simulink model "AGTF30_eng"  (Simulink 8.5)
settings: Solver=FixedStepDiscrete  StartTime=0.0  StopTime=10.0  FixedStep=0.015  RelTol=1e-3  SampleTimeConstraint=STIndependent
model workspace: external: MAT-File (data not in the file)
undefined symbols (not defined in the file or in its folder): MWS, stripchar_TMATS
libraries: Lib_Turbo_StaticCalc_TMATS x6, Lib_Turbo_Compressor_TMATS x3, Lib_Turbo_TurbineNPSS_TMATS x2, Lib_Turbo_Shaft_TMATS x2, Lib_Turbo_Ambient_TMATS x1, Lib_Turbo_Nozzle_TMATS x1, Lib_Turbo_NozzleVar_TMATS x1, Lib_Turbo_Burner_TMATS x1, Lib_Solve_DataOut_TMATS x1, Lib_Turbo_GearBox_TMATS x1, Lib_Turbo_Inlet_TMATS x1, Lib_Turbo_Splitter_TMATS x1
settings Model: Creator=jwchapm2  LastModifiedBy=jwchapm2
settings DataIOCC: ExternalInput=[0 0]  InitialState=[]  SignalLoggingSaveFormat=Dataset  SaveOutput=off  SignalLogging=off  DSMLogging=off  SaveTime=off
settings OptimizationCC: InlineParams=on  BufferReuse=off  ExpressionDepthLimit=128
settings DebuggingCC: UnderspecifiedInitializationDetection=Simplified  MergeDetectMultiDrivingBlocksExec=error  FcnCallInpInsideContextMsg=EnableAllAsError  StateNameClashWarn=none  InitInArrayFormatMsg=none
settings ModelReferenceCC: ModelReferenceNumInstancesAllowed=Single
settings GRTTargetCC: CombineOutputUpdateFcns=on  GRTInterface=off

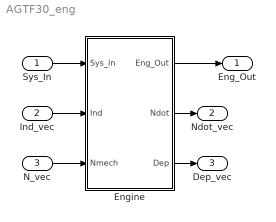
== system AGTF30_eng ==
  Sys_In : Inport
  Ind_vec : Inport  Port=2
  N_vec : Inport  Port=3
  Engine : Subsystem
  Eng_Out : Outport  OutDataTypeStr=Bus: Eng_Bus
  Ndot_vec : Outport  Port=2
  Dep_vec : Outport  Port=3
  wires:
  Sys_In/1 -> Engine/1(Sys_In)
  N_vec/1 -> Engine/3(Nmech)
  Ind_vec/1 -> Engine/2(Ind)
  Engine/3(Dep) -> Dep_vec/1
  Engine/2(Ndot) -> Ndot_vec/1
  Engine/1(Eng_Out) -> Eng_Out/1

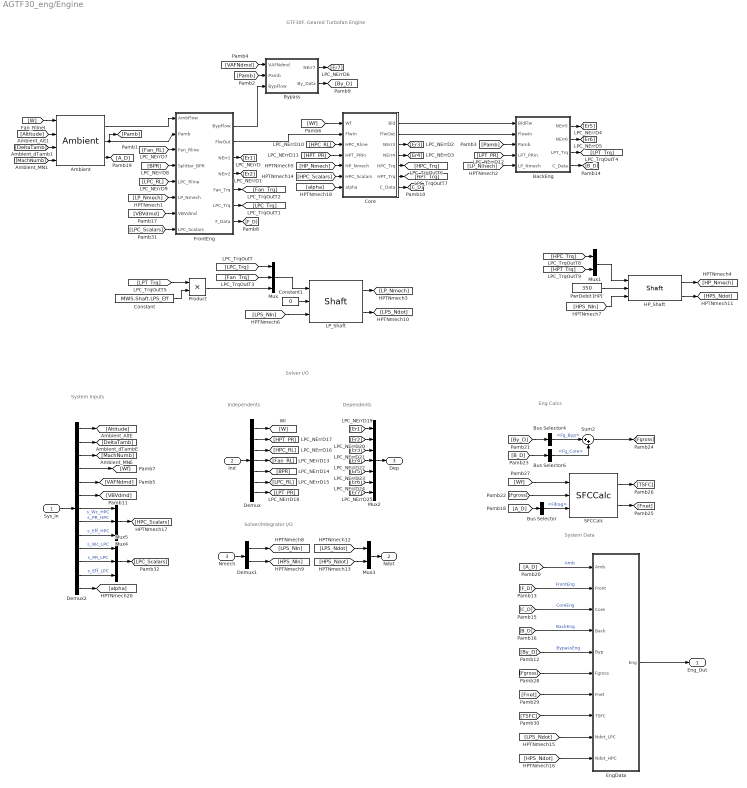
== system AGTF30_eng/Engine ==
  note: GTF30F, Geared Turbofan Engine
  note: System Inputs
  note: Solver I/O
  note: System Data
  note: Solver/Integrator I/O
  note: Independents
  note: Dependents
  note: Eng Calcs
  Sys_In : Inport
  Ind : Inport  Port=2
  Nmech : Inport  Port=3
  Ambient : Lib_Turbo_Ambient_TMATS/Ambient  X_A_AltVec_M=5000*[-1 0 1 2 3 4 5 6 7 8 9 10 12 14 16]  T_A_TsVec_M=[536.51 518.67 500.84 483.03 465.22 447.41 429.62 411.84 394.06 389.97 389.97 389.97 389.97 392.25 397.69]  T_A_PsVec_M=[17.554 14.696 12.228 10.108 8.297 6.759 5.461 4.373 3.468 2.73 2.149 1.692 1.049 0.651 0.406]  AFARc_M=0  X_A_FARVec_M=[0; 0.0050; 0.0100; 0.0150; 0.0200; 0.0250; 0.0300]  T_A_RtArray_M="[0.0686;    0.0686;    0.0686;    0.0686;    0.0686;    0.0686;    0.0686]"  Y_A_TVec_M=[300 10000]  T_A_gammaArray_M=[ 1.4 1.4 1.4 1.4 1.4 1.4 1.4; 1.4 1.4 1.4 1.4 1.4 1.4 1.4]
  BackEng : Subsystem
  Bus Selector : BusSelector  OutputSignals=Fdrag
  Bus Selector4 : BusSelector  OutputSignals=Fg_Byp
  Bus Selector6 : BusSelector  OutputSignals=Fg_Core
  Bypass : Subsystem
  Constant : Constant  Value=MWS.Shaft.LPS_Eff
  Constant1 : Constant  Value=0
  Core : Subsystem
  Demux : Demux  Outputs=7
  Demux1 : Demux  Outputs=2
  Demux2 : Demux  Outputs=13
  EngData : Subsystem
  FrontEng : Subsystem
  HP_Shaft : Lib_Turbo_Shaft_TMATS/Shaft  Shaft_Inertia_M=MWS.Shaft.HPS_Inertia
  LP_Shaft : Lib_Turbo_Shaft_TMATS/Shaft  Shaft_Inertia_M=MWS.Shaft.LPS_Inertia
  Mux : Mux  Inputs=3
  Mux1 : Mux  Inputs=2
  Mux2 : Mux  Inputs=7
  Mux3 : Mux  Inputs=2
  Mux4 : Mux  Inputs=3
  Mux5 : Mux  Inputs=3
  Product : Product
  PwrDebit [HP] : Constant  Value=350
  SFCCalc : Lib_Turbo_SFCCalc_TMATS/SFCCalc
  Sum2 : Sum  Inputs=|++
  Eng_Out : Outport
  Ndot : Outport  Port=2
  Dep : Outport  Port=3
  wires:
  BackEng/4(C_Data) -> [B_D]
  Core/7(C_Data) -> [C_D]
  Ambient/2 -> FrontEng/2(Pamb), [Pamb]
  [W] -> Ambient/1
  [Altitude] -> Ambient/2
  [DeltaTamb] -> Ambient/3
  [MachNumb] -> Ambient/4
  FrontEng/1(BypFlow) -> Bypass/3(BypFlow)
  [Pamb] -> Bypass/2(Pamb)
  FrontEng/2(FlwOut) -> Core/2(FlwIn)
  Core/2(FlwOut) -> BackEng/2(FlowIn)
  Core/1(Bld) -> BackEng/1(BldFlw)
  [Pamb] -> BackEng/3(Pamb)
  FrontEng/6(LPC_Trq) -> [LPC_Trq]
  FrontEng/5(Fan_Trq) -> [Fan_Trq]
  BackEng/3(LPT_Trq) -> [LPT_Trq]
  [LP_Nmech] -> FrontEng/6(LP_Nmech)
  [LP_Nmech] -> BackEng/5(LP_Nmech)
  LP_Shaft/1 -> [LP_Nmech]
  [LPT_Trq] -> Product/1
  [Fan_Trq] -> Mux/2
  [LPC_Trq] -> Mux/1
  Mux/1 -> LP_Shaft/1
  Core/5(HPC_Trq) -> [HPC_Trq]
  Core/6(HPT_Trq) -> [HPT_Trq]
  [HPT_Trq] -> Mux1/2
  [HPC_Trq] -> Mux1/1
  Mux1/1 -> HP_Shaft/1
  HP_Shaft/1 -> [HP_Nmech]
  [HP_Nmech] -> Core/5(HP_Nmech)
  FrontEng/3(NErr1) -> [Er1]
  FrontEng/4(NErr2) -> [Er2]
  Core/3(NErr3) -> [Er3]
  Core/4(NErr4) -> [Er4]
  BackEng/1(NErr5) -> [Er5]
  BackEng/2(NErr6) -> [Er6]
  Bypass/1(NErr7) -> [Er7]
  Demux1/1 -> [LPS_NIn]
  Demux1/2 -> [HPS_NIn]
  [Wf] -> Core/1(Wf)
  [HPS_NIn] -> HP_Shaft/3
  [LPS_NIn] -> LP_Shaft/3
  LP_Shaft/2 -> [LPS_Ndot]
  HP_Shaft/2 -> [HPS_Ndot]
  FrontEng/7(F_Data) -> [F_D]
  [LPC_RL] -> FrontEng/5(LPC_Rline)
  [LPT_PR] -> BackEng/4(LPT_PRIn)
  [BPR] -> FrontEng/4(Splitter_BPR)
  [HPC_RL] -> Core/3(HPC_Rline)
  [Fan_RL] -> FrontEng/3(Fan_Rline)
  [HPT_PR] -> Core/4(HPT_PRIn)
  Ambient/3 -> [A_D]
  Bypass/2(By_Data) -> [By_D]
  Demux/6 -> [LPC_RL]
  Demux/5 -> [BPR]
  Demux/7 -> [LPT_PR]
  Demux/1 -> [W]
  Demux/3 -> [HPC_RL]
  Demux/2 -> [HPT_PR]
  Demux/4 -> [Fan_RL]
  [Er4] -> Mux2/4
  [Er2] -> Mux2/2
  [Er3] -> Mux2/3
  [Er5] -> Mux2/5
  Sys_In/1 -> Demux2/1
  Nmech/1 -> Demux1/1
  [Er1] -> Mux2/1
  Ind/1 -> Demux/1
  [HPS_Ndot] -> Mux3/2
  [LPS_Ndot] -> Mux3/1
  Mux3/1 -> Ndot/1
  [Er6] -> Mux2/6
  Mux2/1 -> Dep/1
  [Er7] -> Mux2/7
  PwrDebit [HP]/1 -> HP_Shaft/2
  [VAFNdmd] -> Bypass/1(VAFNdmd)
  [VBVdmd] -> FrontEng/7(VBVdmd)
  Product/1 -> Mux/3
  Constant/1 -> Product/2
  Ambient/1 -> FrontEng/1(AmbFlow)
  Demux2/5 -> [VAFNdmd]
  Demux2/6 -> [VBVdmd]
  Demux2/1 -> [Altitude]
  Demux2/2 -> [DeltaTamb]
  Demux2/3 -> [MachNumb]
  Demux2/4 -> [Wf]
  [A_D] -> Bus Selector/1
  [By_D] -> Bus Selector4/1
  [B_D] -> Bus Selector6/1
  Bus Selector4/1 -> Sum2/1  "<Fg_Byp>"
  Bus Selector6/1 -> Sum2/2  "<Fg_Core>"
  Sum2/1 -> [Fgross]
  [A_D] -> EngData/1(Amb)  "Amb"
  [F_D] -> EngData/2(Front)  "FrontEng"
  [C_D] -> EngData/3(Core)  "CoreEng"
  [B_D] -> EngData/4(Back)  "BackEng"
  [By_D] -> EngData/5(Byp)  "BypassEng"
  [Fnet] -> EngData/7(Fnet)
  [Fgross] -> EngData/6(Fgross)
  [HPS_Ndot] -> EngData/10(Ndot_HPC)
  [LPS_Ndot] -> EngData/9(Ndot_LPC)
  Bus Selector/1 -> SFCCalc/3  "<Fdrag>"
  [Fgross] -> SFCCalc/2
  SFCCalc/2 -> [Fnet]
  SFCCalc/1 -> [TSFC]
  [Wf] -> SFCCalc/1
  [TSFC] -> EngData/8(TSFC)
  Constant1/1 -> LP_Shaft/2
  [HPC_Scalars] -> Core/6(HPC_Scalars)
  [LPC_Scalars] -> FrontEng/8(LPC_Scalars)
  Mux4/1 -> [HPC_Scalars]
  Mux5/1 -> [LPC_Scalars]
  Demux2/8 -> Mux4/2  "s_PR_HPC"
  Demux2/7 -> Mux4/1  "s_Wc_HPC"
  Demux2/9 -> Mux4/3  "s_Eff_HPC"
  Demux2/10 -> Mux5/1  "s_Wc_LPC"
  Demux2/11 -> Mux5/2  "s_PR_LPC"
  Demux2/12 -> Mux5/3  "s_Eff_LPC"
  EngData/1(Eng) -> Eng_Out/1
  [alpha] -> Core/7(alpha)
  Demux2/13 -> [alpha]

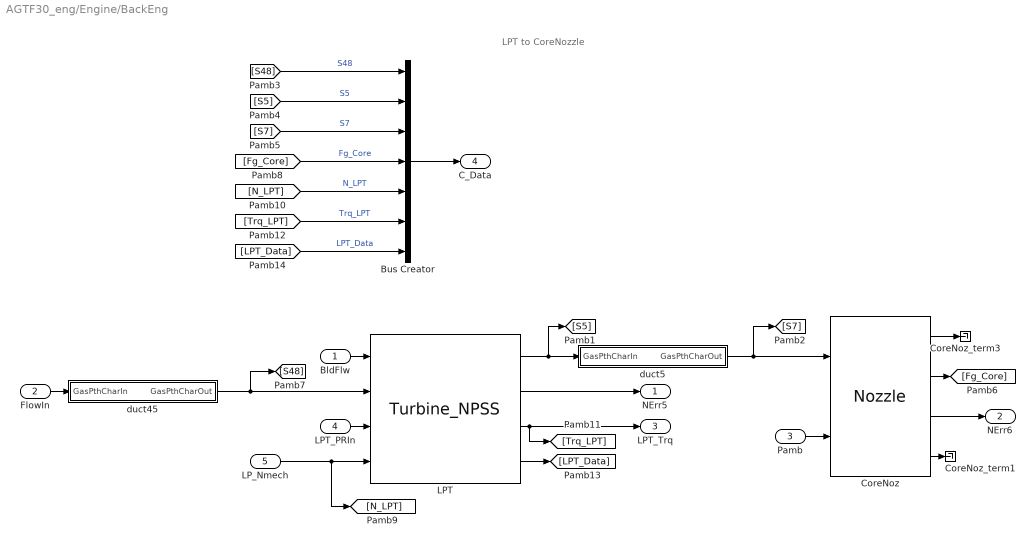
== system AGTF30_eng/Engine/BackEng ==
  note: LPT to CoreNozzle
  BldFlw : Inport
  FlowIn : Inport  Port=2
  Pamb : Inport  Port=3
  LPT_PRIn : Inport  Port=4
  LP_Nmech : Inport  Port=5
  Bus Creator : BusCreator  Inputs=7
  CoreNoz : Lib_Turbo_Nozzle_TMATS/Nozzle  SWType_M=Convergent  N_TArea_M=MWS.NozCor.Ath  N_EArea_M=110.7  N_FL_M=0.00  X_N_TtVec2_M=[300 10000]  T_N_TGArray_M=[1 1]  X_N_PEQPaVec_M=[0 10000]  T_N_CdThArray_M=[1 1]  T_N_CvArray_M=[1 1]  CfgEn_M=on  T_N_CfgArray_M=[1 1]*MWS.NozCor.Cfg  X_N_FARVec_M=[0; 0.0050; 0.0100; 0.0150; 0.0200; 0.0250; 0.0300]  T_N_RtArray_M="[0.0686;    0.0686;    0.0686;    0.0686;    0.0686;    0.0686;    0.0686]"  Y_N_TtVec_M=[300 10000]  T_N_MAP_gammaArray_M=[ 1.4 1.4 1.4 1.4 1.4 1.4 1.4; 1.4 1.4 1.4 1.4 1.4 1.4 1.4]  iDesign_M=2  WDes_M=MWS.NozCor.WDes  FVar_M=strcat('iDes_',stripchar_TMATS(gcb),'.bin')
  CoreNoz_term1 : Terminator
  CoreNoz_term3 : Terminator
  LPT : Lib_Turbo_TurbineNPSS_TMATS/Turbine_NPSS  X_T_Map_PRVec_M=MWS.LPT.PRVec  Y_T_Map_NcVec_M=MWS.LPT.NcVec  T_T_Map_WcArray_M=MWS.LPT.WcArray  T_T_Map_EffArray_M=MWS.LPT.effArray  s_T_Nc_M=MWS.LPT.s_Nc  s_T_Wc_M=MWS.LPT.s_Wc  s_T_PR_M=MWS.LPT.s_PR  s_T_Eff_M=MWS.LPT.s_Eff  ConfigNPSS_M=1  Scale_M=none  CFlwEn_M=on  T_CoolFlwPos_M=MWS.LPT.CWPos  iDesign_M=2  NcDes_M=MWS.LPT.NcMapDes  EffDes_M=MWS.LPT.EffDes  PRDes_M=MWS.LPT.PRMapDes  NDes_M=MWS.LPT.NDes  FVar_M=strcat('iDes_',stripchar_TMATS(gcb),'.bin')  BlkNm_M=double(gcb)  HP_M=off
  duct45 : Subsystem  mask(T-MATS: Duct Library Block){dP_M=MWS.Duct.D45, MNdes_M=MWS.Duct.MNdes45, Ath_M=MWS.Duct.Ath45}
      mask prompts: dP_M "dP_M - Delta Pressure [frac lost]"; MNdes_M "MNdes_M - Mach Number Design"; Ath_M "Ath_M - Throat Area [in2]"
      mask help: This block simulates the performance of a duct using basic fluid dynamic equations and properties.
      mask Help: web(which('Turbo_TMATS_Dct.html'),'-helpbrowser')
  duct5 : Subsystem  mask(T-MATS: Duct Library Block){dP_M=MWS.Duct.D5, MNdes_M=MWS.Duct.MNdes5, Ath_M=MWS.Duct.Ath5}
      mask prompts: dP_M "dP_M - Delta Pressure [frac lost]"; MNdes_M "MNdes_M - Mach Number Design"; Ath_M "Ath_M - Throat Area [in2]"
      mask help: This block simulates the performance of a duct using basic fluid dynamic equations and properties.
      mask Help: web(which('Turbo_TMATS_Dct.html'),'-helpbrowser')
  NErr5 : Outport
  NErr6 : Outport  Port=2
  LPT_Trq : Outport  Port=3
  C_Data : Outport  Port=4
  wires:
  duct5/1(GasPthCharOut) -> [S7], CoreNoz/1
  LPT/2 -> NErr5/1
  LPT/3 -> [Trq_LPT], LPT_Trq/1
  Pamb/1 -> CoreNoz/2
  LP_Nmech/1 -> [N_LPT], LPT/4
  CoreNoz/2 -> [Fg_Core]
  CoreNoz/4 -> CoreNoz_term1/1
  FlowIn/1 -> duct45/1(GasPthCharIn)
  duct45/1(GasPthCharOut) -> [S48], LPT/2
  LPT/1 -> duct5/1(GasPthCharIn), [S5]
  CoreNoz/1 -> CoreNoz_term3/1
  CoreNoz/3 -> NErr6/1
  LPT_PRIn/1 -> LPT/3
  BldFlw/1 -> LPT/1
  Bus Creator/1 -> C_Data/1
  [S5] -> Bus Creator/2  "S5"
  [S7] -> Bus Creator/3  "S7"
  [S48] -> Bus Creator/1  "S48"
  [Fg_Core] -> Bus Creator/4  "Fg_Core"
  [N_LPT] -> Bus Creator/5  "N_LPT"
  [Trq_LPT] -> Bus Creator/6  "Trq_LPT"
  LPT/4 -> [LPT_Data]
  [LPT_Data] -> Bus Creator/7  "LPT_Data"

== system AGTF30_eng/Engine/Bypass ==
  VAFNdmd : Inport
  Pamb : Inport  Port=2
  BypFlow : Inport  Port=3
  Bus Creator : BusCreator  Inputs=2
  BypNoz : Lib_Turbo_NozzleVar_TMATS/NozzleVar  SWType_M=1  N_FL_M=0.00  X_N_TtVec2_M=[300 10000]  T_N_TGArray_M=[1 1]  X_N_PEQPaVec_M=[0 10000]  T_N_CdThArray_M=[1 1]  T_N_CvArray_M=[1 1]  CfgEn_M=on  T_N_CfgArray_M=[1 1]* MWS.NozByp.Cfg  X_N_FARVec_M=[0; 0.0050; 0.0100; 0.0150; 0.0200; 0.0250; 0.0300]  T_N_RtArray_M="[0.0686;    0.0686;    0.0686;    0.0686;    0.0686;    0.0686;    0.0686]"  Y_N_TtVec_M=[300 10000]  T_N_MAP_gammaArray_M=[ 1.4 1.4 1.4 1.4 1.4 1.4 1.4; 1.4 1.4 1.4 1.4 1.4 1.4 1.4]  iDesign_M=2  WDes_M=MWS.NozByp.WDes  FVar_M=strcat('iDes_',stripchar_TMATS(gcb),'.bin')  N_TArea_M=0  N_EArea_M=0
  BypNoz_term1 : Terminator
  BypNoz_term3 : Terminator
  duct17 : Subsystem  mask(T-MATS: Duct Library Block){dP_M=MWS.Duct.D17, MNdes_M=MWS.Duct.MNdes17, Ath_M=MWS.Duct.Ath17}
      mask prompts: dP_M "dP_M - Delta Pressure [frac lost]"; MNdes_M "MNdes_M - Mach Number Design"; Ath_M "Ath_M - Throat Area [in2]"
      mask help: This block simulates the performance of a duct using basic fluid dynamic equations and properties.
      mask Help: web(which('Turbo_TMATS_Dct.html'),'-helpbrowser')
  NErr7 : Outport
  By_Data : Outport  Port=2
  wires:
  BypNoz/1 -> BypNoz_term3/1
  BypNoz/4 -> BypNoz_term1/1
  Pamb/1 -> BypNoz/2
  BypNoz/2 -> [Fg_Byp]
  BypNoz/3 -> NErr7/1
  BypFlow/1 -> duct17/1(GasPthCharIn)
  duct17/1(GasPthCharOut) -> BypNoz/1, [S17]
  [S17] -> Bus Creator/1  "S17"
  Bus Creator/1 -> By_Data/1
  [Fg_Byp] -> Bus Creator/2  "Fg_Byp"
  VAFNdmd/1 -> BypNoz/3, BypNoz/4

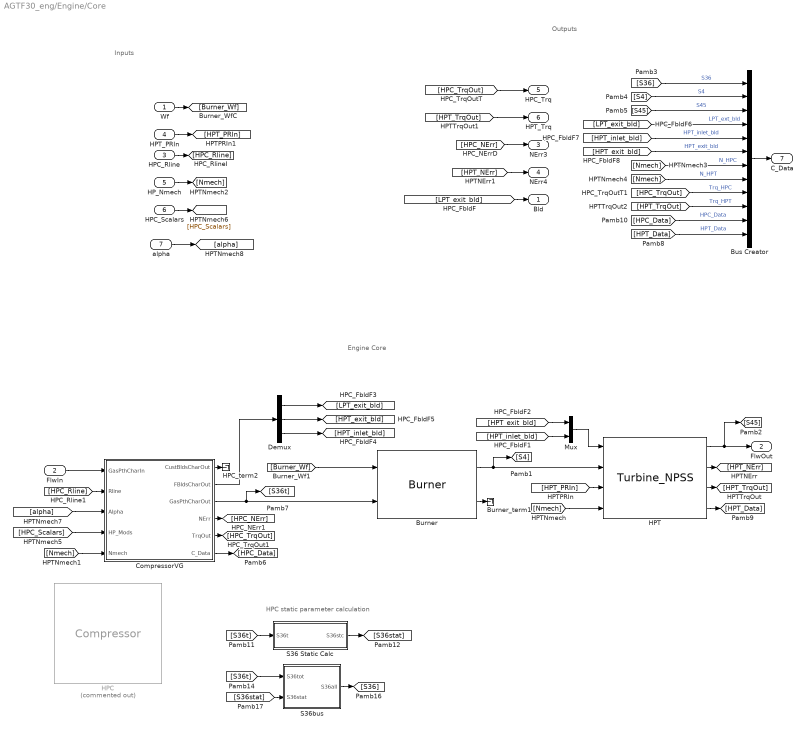
== system AGTF30_eng/Engine/Core ==
  note: HPC static parameter calculation
  note: Engine Core
  note: Inputs
  note: Outputs
  Wf : Inport
  FlwIn : Inport  Port=2
  HPC_Rline : Inport  Port=3
  HPT_PRIn : Inport  Port=4
  HP_Nmech : Inport  Port=5
  HPC_Scalars : Inport  Port=6
  alpha : Inport  Port=7
  Burner : Lib_Turbo_Burner_TMATS/Burner  LHVEn_M=on  LHV_M=MWS.Burn.LHV  Eff_M=MWS.Burn.Eff  hFuel_M=-1200  dPnormBurner_M=MWS.Burn.dPqP_dmd
  Burner_term1 : Terminator
  Bus Creator : BusCreator  Inputs=12
  CompressorVG : Subsystem  mask(T-MATS: CompressorVG Library Block){X_C_RlineVec_M=MWS.HPC.RVec, Z_C_AlphaVec_M=MWS.HPC.Alpha, Y_C_Map_NcVec_M=MWS.HPC.NcVec, T_C_Map_WcArray_M=MWS.HPC.WcMap, T_C_Map_PRArray_M=MWS.HPC.PRMap, T_C_Map_EffArray_M=MWS.HPC.EffMap, s_C_Nc_M=MWS.HPC.s_Nc, s_C_Wc_M=MWS.HPC.s_Wc, s_C_PR_M=MWS.HPC.s_PR, s_C_Eff_M=MWS.HPC.s_Eff, SL_M=off, Scale_M=none, CBLDEN_M=off, C_CBD_M=0, C_CBFht_M=0.5, C_CBFPt_M=0.5, FBLDEN_M=on, C_FBD_M=MWS.HPC.FBD, C_BFht_M=MWS.HPC.BFht, C_BFPt_M=MWS.HPC.BFPt, DefSMEn_M=off, SMNEn_M=off, SRline_M=1, X_C_Map_WcSurgeVec_M=MWS.HPC.WcSM, T_C_Map_PRSurgeVec_M=MWS.HPC.PRSM, iDesign_M=2, NcDes_M=10000, EffDes_M=0.95, PRDes_M=20, RlineDes_M=2, FVar_M=strcat('iDes_',stripchar_TMATS(gcb),'.bin'), BlkNm_M=double(gcb), HP_M=on}
      mask prompts: X_C_RlineVec_M "X_C_RlineVec_M - Compressor Map Rline Vector (X-axis)(nx1)"; Z_C_AlphaVec_M "Z_C_Map_AlphaVec_M - Compressor Alpha Vector (Z-axis)(rx1)"; Y_C_Map_NcVec_M "Y_C_Map_NcVec_M - Compressor Map Corrected Speed Vector (Y-axis)(mx1)"; T_C_Map_WcArray_M "T_C_Map_WcArray_M - Compressor Map Flow Array (Wc = f(Nc, Rline,Alpha))(mxnxr)"; T_C_Map_PRArray_M "T_C_Map_PRArray_M - Compressor Map Pressure Ratio Array (PR = f(Nc, Rline,Alpha))(mxnxr)"; T_C_Map_EffArray_M "T_C_Map_EffArray_M - Compressor Map Efficiency Array (Eff = f(Nc, Rline,Alpha)(mxnxr)"; s_C_Nc_M "s_C_Nc_M - Corrected Speed Scalar Constant (C_Nc)"; s_C_Wc_M "s_C_Wc_M - Flow Scalar Constant (C_Wc)"; s_C_PR_M "s_C_PR_M - Pressure Ratio Scalar Constant (C_PR)"; s_C_Eff_M "s_C_Eff_M - Efficiency Scalar Constant (C_Eff)"; SL_M "Include surge line"; Scale_M "Scalars"; CBLDEN_M "CBLDEN_M - Customer Bleed Enable [0 - off, 1 - on]"; C_CBD_M "C_CBD_M - Customer or Flow based Bleed Demand[pps] (cbx1)"; C_CBFht_M "C_CBFht_M - Customer or Flow based Bleed Fractional enthalpy[frac] (cbx1)"; C_CBFPt_M "C_CBFPt_M - Customer or Flow based Bleed Fractional Total Pressure[frac] (cbx1)"; FBLDEN_M "FBLDEN_M - Fractional Bleed Enable [0 - off, 1 - on]"; C_FBD_M "C_FBD_M - Fractional Bleed Demand[frac] (bx1)"; C_BFht_M "C_BFht_M - Engine Bleed Fractional Enthalpy[frac] (bx1)"; C_BFPt_M "C_BFPt_M - Engine Bleed Fractional Total Pressure[frac] (bx1)"; DefSMEn_M "DefSMEn_M - Use map default (Rline = 1) surge line"; SMNEn_M "SMNEn_M - Use constant Nc-based instead of constant Wc-based surge margin calculation"; SRline_M "SRline_M - Rline defined as surge line"; X_C_Map_WcSurgeVec_M "X_C_Map_WcSurgeVec_M - map Compensated flow surge vector (Vec = f(Alpha)) (sxr)"; T_C_Map_PRSurgeVec_M "T_C_Map_PRSurgeVec_M - map Surge Line Pressure Ratio vector (Vec = f(Alpha)) (sxr)"; iDesign_M "iDesign_M - Design fork (0 - Enable iDes, 1 - Use iDes Scalars, 2 - Use Specified Input Scalars)"; NcDes_M "NcDes_M - map Design Corrected Shaft Speed [rpm]"; EffDes_M "EffDes_M  - Design Efficiency [frac]"; PRDes_M "PRDes_M - Design Pressure Ratio [frac]"; RlineDes_M "RlineDes_M - map Design Rline"; FVar_M "FVar_M - File name for iDes Variables"; BlkNm_M "Block name as double for Simulink output"; HP_M "HP_M - Enable Health Parameter input (3x1 vector)"
      mask help:
      | This block simulates the performance of a compressor using basic thermodynamic equations, properties, and table lookups.
      |
      | This block also takes into account 3 dimensional performance maps. Shifting between the tables can be completed using the Alpha term. This feature can be used for simulation of variable geometries.
      mask init:
      | MSK_CompInit_TMATS
      mask Help: web(which('Turbo_TMATS_CmpVG.html'),'-helpbrowser')
      mask TypeOptions Scale_M: none | user defined | iDesign
      mask Callback CBLDEN_M: MSK_SEC_Enables_TMATS('CBLDEN_M',[14 15 16],'en')
      mask Callback FBLDEN_M: MSK_SEC_Enables_TMATS('FBLDEN_M',[18 19 20],'en')
      mask Callback DefSMEn_M:
      | MSK_SEC_Enables_TMATS('DefSMEn_M',[24 25],'dis')
      | MSK_SEC_Enables_TMATS('DefSMEn_M',[23],'en')
      mask Callback iDesign_M:
      | MSK_SEC_Enables_Ides_TMATS('iDesign_M',[7 8 9 10],'G1')
      | MSK_SEC_Enables_Ides_TMATS('iDesign_M',[27 28 29 30],'G2')
      | MSK_SEC_Enables_Ides_TMATS('iDesign_M',[31],'G3')
      mask DialogControl Control2 Prompt: Plot Map
      mask DialogControl Control2 Callback: MSK_PlotCMap_TMATS()
  Demux : Demux  Outputs=3
  HPC : Lib_Turbo_Compressor_TMATS/Compressor  Commented=on  X_C_RlineVec_M=MWS.HPC.RVec  Z_C_AlphaVec_M=1  Y_C_Map_NcVec_M=MWS.HPC.NcVec  T_C_Map_WcArray_M=MWS.HPC.WcArray  T_C_Map_PRArray_M=MWS.HPC.PRArray  T_C_Map_EffArray_M=MWS.HPC.EffArray  s_C_Nc_M=MWS.HPC.s_Nc  s_C_Wc_M=MWS.HPC.s_Wc  s_C_PR_M=MWS.HPC.s_PR  s_C_Eff_M=MWS.HPC.s_Eff  SL_M=off  Scale_M=none  CBLDEN_M=off  C_CBD_M=0  C_CBFht_M=0.5  C_CBFPt_M=0.5  FBLDEN_M=on  C_FBD_M=MWS.HPC.FBD  C_BFht_M=MWS.HPC.BFht  C_BFPt_M=MWS.HPC.BFPt  DefSMEn_M=off  SMNEn_M=off  SRline_M=1  X_C_Map_WcSurgeVec_M=MWS.HPC.SM_WcVec  T_C_Map_PRSurgeVec_M=MWS.HPC.SM_PRVec  iDesign_M=2  NcDes_M=MWS.HPC.NcDesMap  EffDes_M=MWS.HPC.EffDes  PRDes_M=MWS.HPC.PRDes  RlineDes_M=MWS.HPC.RlineDesMap  FVar_M=strcat('iDes_',stripchar_TMATS(gcb),'.bin')  BlkNm_M=double(gcb)  HP_M=on
  HPC_term2 : Terminator
  HPT : Lib_Turbo_TurbineNPSS_TMATS/Turbine_NPSS  X_T_Map_PRVec_M=MWS.HPT.PRVec  Y_T_Map_NcVec_M=MWS.HPT.NcVec  T_T_Map_WcArray_M=MWS.HPT.WcArray  T_T_Map_EffArray_M=MWS.HPT.effArray  s_T_Nc_M=MWS.HPT.s_Nc  s_T_Wc_M=MWS.HPT.s_Wc  s_T_PR_M=MWS.HPT.s_PR  s_T_Eff_M=MWS.HPT.s_Eff  ConfigNPSS_M=1  Scale_M=none  CFlwEn_M=on  T_CoolFlwPos_M=MWS.HPT.CWPos  iDesign_M=2  NcDes_M=MWS.HPT.NcMapDes  EffDes_M=MWS.HPT.EffDes  PRDes_M=MWS.HPT.PRMapDes  NDes_M=MWS.HPT.NDes  FVar_M=strcat('iDes_',stripchar_TMATS(gcb),'.bin')  BlkNm_M=double(gcb)  HP_M=off
  Mux : Mux  Inputs=2
  S36 Static Calc : Subsystem
  S36bus : Subsystem
  Bld : Outport
  FlwOut : Outport  Port=2
  NErr3 : Outport  Port=3
  NErr4 : Outport  Port=4
  HPC_Trq : Outport  Port=5
  HPT_Trq : Outport  Port=6
  C_Data : Outport  Port=7
  wires:
  Burner/1 -> [S4], HPT/2
  HP_Nmech/1 -> [Nmech]
  [Nmech] -> CompressorVG/5(Nmech)
  HPT/3 -> [HPT_TrqOut]
  [Nmech] -> HPT/4
  Wf/1 -> [Burner_Wf]
  HPT/4 -> [HPT_Data]
  [HPT_PRIn] -> HPT/3
  [HPC_TrqOut] -> HPC_Trq/1
  [HPC_Rline] -> CompressorVG/2(Rline)
  CompressorVG/4(NErr) -> [HPC_NErr]
  FlwIn/1 -> CompressorVG/1(GasPthCharIn)
  HPT/1 -> [S45], FlwOut/1
  [HPC_NErr] -> NErr3/1
  HPC_Rline/1 -> [HPC_Rline]
  HPT/2 -> [HPT_NErr]
  CompressorVG/1(CustBldsCharOut) -> HPC_term2/1
  CompressorVG/6(C_Data) -> [HPC_Data]
  CompressorVG/5(TrqOut) -> [HPC_TrqOut]
  [LPT_exit_bld] -> Bld/1
  CompressorVG/3(GasPthCharOut) -> [S36t], Burner/2
  Burner/2 -> Burner_term1/1
  [HPT_TrqOut] -> HPT_Trq/1
  [HPT_NErr] -> NErr4/1
  HPT_PRIn/1 -> [HPT_PRIn]
  [S36] -> Bus Creator/1  "S36"
  [HPT_inlet_bld] -> Bus Creator/5  "HPT_inlet_bld"
  [S45] -> Bus Creator/3  "S45"
  [S4] -> Bus Creator/2  "S4"
  [HPT_exit_bld] -> Bus Creator/6  "HPT_exit_bld"
  [LPT_exit_bld] -> Bus Creator/4  "LPT_ext_bld"
  Bus Creator/1 -> C_Data/1
  [Nmech] -> Bus Creator/7  "N_HPC"
  [Nmech] -> Bus Creator/8  "N_HPT"
  [HPC_TrqOut] -> Bus Creator/9  "Trq_HPC"
  [HPT_TrqOut] -> Bus Creator/10  "Trq_HPT"
  CompressorVG/2(FBldsCharOut) -> Demux/1
  Demux/1 -> [LPT_exit_bld]
  Demux/2 -> [HPT_exit_bld]
  Demux/3 -> [HPT_inlet_bld]
  [HPT_inlet_bld] -> Mux/2
  [HPT_exit_bld] -> Mux/1
  Mux/1 -> HPT/1
  [Burner_Wf] -> Burner/1
  [HPC_Data] -> Bus Creator/11  "HPC_Data"
  [HPT_Data] -> Bus Creator/12  "HPT_Data"
  [S36t] -> S36 Static Calc/1(S36t)
  S36 Static Calc/1(S36stc) -> [S36stat]
  [S36t] -> S36bus/1(S36tot)
  [S36stat] -> S36bus/2(S36stat)
  S36bus/1(S36all) -> [S36]
  [HPC_Scalars] -> CompressorVG/4(HP_Mods)
  HPC_Scalars/1 -> [HPC_Scalars]
  [alpha] -> CompressorVG/3(Alpha)
  alpha/1 -> [alpha]

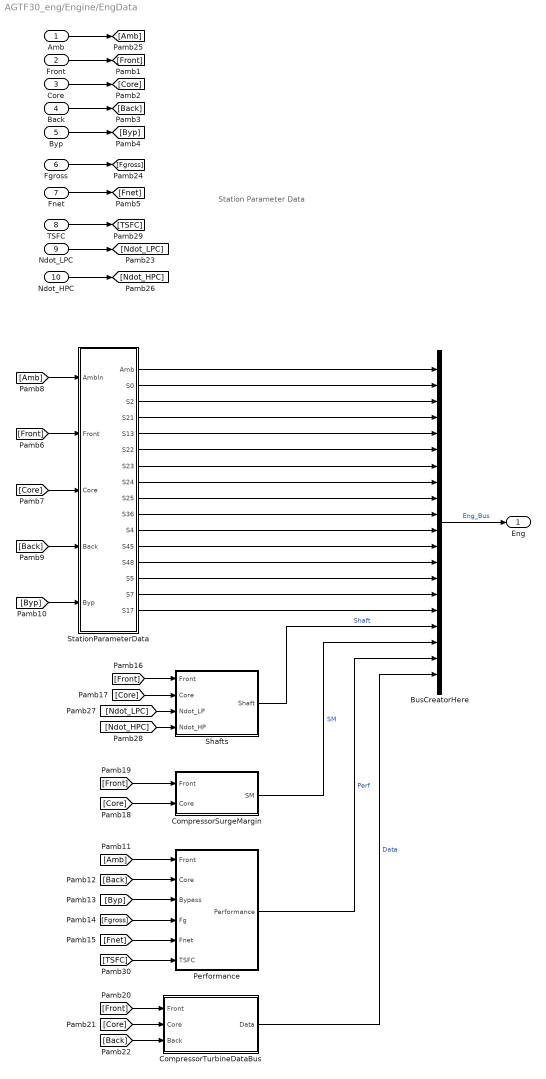
== system AGTF30_eng/Engine/EngData ==
  note: Station Parameter Data
  Amb : Inport
  Front : Inport  Port=2
  Core : Inport  Port=3
  Back : Inport  Port=4
  Byp : Inport  Port=5
  Fgross : Inport  Port=6
  Fnet : Inport  Port=7
  TSFC : Inport  Port=8
  Ndot_LPC : Inport  Port=9
  Ndot_HPC : Inport  Port=10
  BusCreatorHere : BusCreator  Inputs=20
  CompressorSurgeMargin : Subsystem
  CompressorTurbineDataBus : Subsystem
  Performance : Subsystem
  Shafts : Subsystem
  StationParameterData : Subsystem
  Eng : Outport
  wires:
  BusCreatorHere/1 -> Eng/1  "Eng_Bus"
  Amb/1 -> [Amb]
  Front/1 -> [Front]
  Core/1 -> [Core]
  Back/1 -> [Back]
  Byp/1 -> [Byp]
  Fgross/1 -> [Fgross]
  Fnet/1 -> [Fnet]
  [Amb] -> StationParameterData/1(AmbIn)
  [Front] -> StationParameterData/2(Front)
  [Core] -> StationParameterData/3(Core)
  [Back] -> StationParameterData/4(Back)
  [Byp] -> StationParameterData/5(Byp)
  [Front] -> CompressorTurbineDataBus/1(Front)
  [Core] -> CompressorTurbineDataBus/2(Core)
  [Back] -> CompressorTurbineDataBus/3(Back)
  [Front] -> CompressorSurgeMargin/1(Front)
  [Core] -> CompressorSurgeMargin/2(Core)
  [Amb] -> Performance/1(Front)
  [Back] -> Performance/2(Core)
  [Byp] -> Performance/3(Bypass)
  [Fgross] -> Performance/4(Fg)
  [Fnet] -> Performance/5(Fnet)
  [Front] -> Shafts/1(Front)
  [Core] -> Shafts/2(Core)
  Shafts/1(Shaft) -> BusCreatorHere/17  "Shaft"
  StationParameterData/4(S21) -> BusCreatorHere/4
  StationParameterData/9(S25) -> BusCreatorHere/9
  StationParameterData/6(S22) -> BusCreatorHere/6
  StationParameterData/10(S36) -> BusCreatorHere/10
  StationParameterData/8(S24) -> BusCreatorHere/8
  StationParameterData/11(S4) -> BusCreatorHere/11
  StationParameterData/1(Amb) -> BusCreatorHere/1
  StationParameterData/3(S2) -> BusCreatorHere/3
  StationParameterData/2(S0) -> BusCreatorHere/2
  StationParameterData/13(S48) -> BusCreatorHere/13
  StationParameterData/12(S45) -> BusCreatorHere/12
  StationParameterData/15(S7) -> BusCreatorHere/15
  StationParameterData/16(S17) -> BusCreatorHere/16
  StationParameterData/14(S5) -> BusCreatorHere/14
  StationParameterData/5(S13) -> BusCreatorHere/5
  StationParameterData/7(S23) -> BusCreatorHere/7
  CompressorSurgeMargin/1(SM) -> BusCreatorHere/18  "SM"
  Performance/1(Performance) -> BusCreatorHere/19  "Perf"
  CompressorTurbineDataBus/1(Data) -> BusCreatorHere/20  "Data"
  Ndot_LPC/1 -> [Ndot_LPC]
  Ndot_HPC/1 -> [Ndot_HPC]
  [Ndot_LPC] -> Shafts/3(Ndot_LP)
  [Ndot_HPC] -> Shafts/4(Ndot_HP)
  TSFC/1 -> [TSFC]
  [TSFC] -> Performance/6(TSFC)

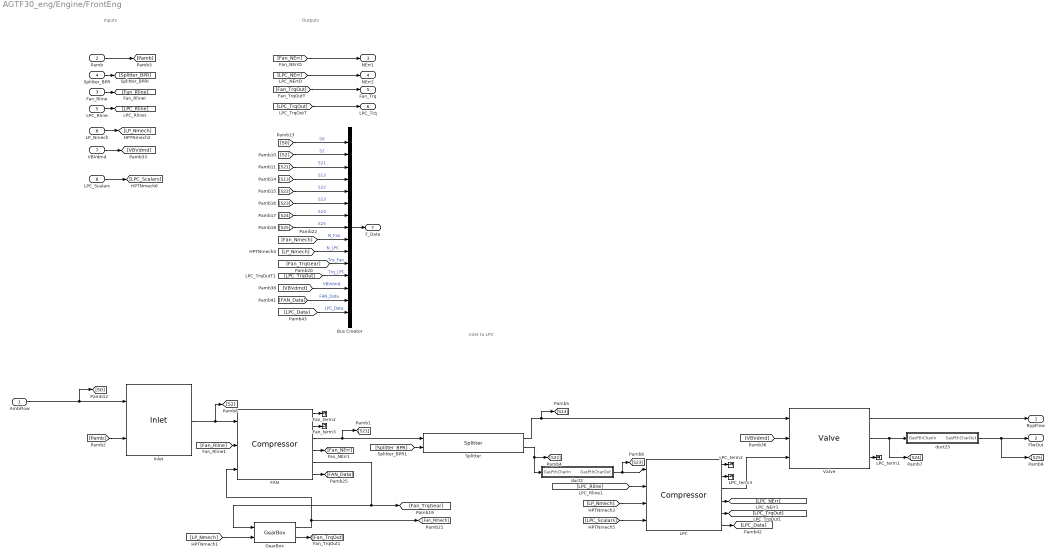
== system AGTF30_eng/Engine/FrontEng ==
  note: Inlet to LPC
  note: Inputs
  note: Outputs
  AmbFlow : Inport
  Pamb : Inport  Port=2
  Fan_Rline : Inport  Port=3
  Splitter_BPR : Inport  Port=4
  LPC_Rline : Inport  Port=5
  LP_Nmech : Inport  Port=6
  VBVdmd : Inport  Port=7
  LPC_Scalars : Inport  Port=8
  Bus Creator : BusCreator  Inputs=15
  FAN : Lib_Turbo_Compressor_TMATS/Compressor  X_C_RlineVec_M=MWS.FAN.RVec  Z_C_AlphaVec_M=1  Y_C_Map_NcVec_M=MWS.FAN.NcVec  T_C_Map_WcArray_M=MWS.FAN.WcArray  T_C_Map_PRArray_M=MWS.FAN.PRArray  T_C_Map_EffArray_M=MWS.FAN.EffArray  s_C_Nc_M=MWS.FAN.s_Nc  s_C_Wc_M=MWS.FAN.s_Wc  s_C_PR_M=MWS.FAN.s_PR  s_C_Eff_M=MWS.FAN.s_Eff  SL_M=off  Scale_M=none  CBLDEN_M=off  C_CBD_M=0  C_CBFht_M=0.5  C_CBFPt_M=0.5  FBLDEN_M=off  C_FBD_M=0  C_BFht_M=0.5  C_BFPt_M=0.5  DefSMEn_M=off  SMNEn_M=off  SRline_M=1  X_C_Map_WcSurgeVec_M=MWS.FAN.SM_WcVec  T_C_Map_PRSurgeVec_M=MWS.FAN.SM_PRVec  iDesign_M=2  NcDes_M=MWS.FAN.NcDesMap  EffDes_M=MWS.FAN.EffDes  PRDes_M=MWS.FAN.PRDes  RlineDes_M=MWS.FAN.RlineDesMap  FVar_M=strcat('iDes_',stripchar_TMATS(gcb),'.bin')  BlkNm_M=double(gcb)  HP_M=off
  Fan_term2 : Terminator
  Fan_term3 : Terminator
  GearBox : Lib_Turbo_GearBox_TMATS/GearBox  R_M=MWS.GearBox.GearRatio  Eff_M=MWS.GearBox.Eff
  Inlet : Lib_Turbo_Inlet_TMATS/Inlet  eRambase_M=MWS.Inlet.eRam  X_eRamVec_M=MWS.Inlet.eRamVec  T_eRamtbl_M=MWS.Inlet.eRamTBL
  LPC : Lib_Turbo_Compressor_TMATS/Compressor  X_C_RlineVec_M=MWS.LPC.RVec  Z_C_AlphaVec_M=1  Y_C_Map_NcVec_M=MWS.LPC.NcVec  T_C_Map_WcArray_M=MWS.LPC.WcArray  T_C_Map_PRArray_M=MWS.LPC.PRArray  T_C_Map_EffArray_M=MWS.LPC.EffArray  s_C_Nc_M=MWS.LPC.s_Nc  s_C_Wc_M=MWS.LPC.s_Wc  s_C_PR_M=MWS.LPC.s_PR  s_C_Eff_M=MWS.LPC.s_Eff  SL_M=on  Scale_M=none  CBLDEN_M=off  C_CBD_M=0  C_CBFht_M=0.5  C_CBFPt_M=0.5  FBLDEN_M=off  C_FBD_M=0  C_BFht_M=0.5  C_BFPt_M=0.5  DefSMEn_M=off  SMNEn_M=off  SRline_M=1  X_C_Map_WcSurgeVec_M=MWS.LPC.SM_WcVec  T_C_Map_PRSurgeVec_M=MWS.LPC.SM_PRVec  iDesign_M=2  NcDes_M=MWS.LPC.NcDesMap  EffDes_M=MWS.LPC.EffDes  PRDes_M=MWS.LPC.PRDes  RlineDes_M=MWS.LPC.RlineDesMap  FVar_M=strcat('iDes_',stripchar_TMATS(gcb),'.bin')  BlkNm_M=double(gcb)  HP_M=on
  LPC_term1 : Terminator
  LPC_term2 : Terminator
  LPC_term3 : Terminator
  Splitter : Lib_Turbo_Splitter_TMATS/Splitter
  Valve : Lib_Turbo_Valve_TMATS/Valve  VFO_M=MWS.VBV.fullopen  VDZ_M=MWS.VBV.fullclosed  VAe_M=MWS.VBV.Ae  X_VPRVec_M=MWS.VBV.PRVec  T_VWArray_M=MWS.VBV.Flowe
  duct2 : Subsystem  mask(T-MATS: Duct Library Block){dP_M=MWS.Duct.D2, MNdes_M=MWS.Duct.MNdes2, Ath_M=MWS.Duct.Ath2}
      mask prompts: dP_M "dP_M - Delta Pressure [frac lost]"; MNdes_M "MNdes_M - Mach Number Design"; Ath_M "Ath_M - Throat Area [in2]"
      mask help: This block simulates the performance of a duct using basic fluid dynamic equations and properties.
      mask Help: web(which('Turbo_TMATS_Dct.html'),'-helpbrowser')
  duct25 : Subsystem  mask(T-MATS: Duct Library Block){dP_M=MWS.Duct.D25, MNdes_M=MWS.Duct.MNdes25, Ath_M=MWS.Duct.Ath25}
      mask prompts: dP_M "dP_M - Delta Pressure [frac lost]"; MNdes_M "MNdes_M - Mach Number Design"; Ath_M "Ath_M - Throat Area [in2]"
      mask help: This block simulates the performance of a duct using basic fluid dynamic equations and properties.
      mask Help: web(which('Turbo_TMATS_Dct.html'),'-helpbrowser')
  BypFlow : Outport
  FlwOut : Outport  Port=2
  NErr1 : Outport  Port=3
  NErr2 : Outport  Port=4
  Fan_Trq : Outport  Port=5
  LPC_Trq : Outport  Port=6
  F_Data : Outport  Port=7
  wires:
  [Splitter_BPR] -> Splitter/2
  GearBox/2 -> [Fan_TrqOut]
  FAN/3 -> [S21], Splitter/1
  GearBox/1 -> FAN/3, [Fan_Nmech]
  Splitter/2 -> [S22], duct2/1(GasPthCharIn)
  Fan_Rline/1 -> [Fan_Rline]
  FAN/2 -> Fan_term3/1
  [Fan_TrqOut] -> Fan_Trq/1
  FAN/6 -> [FAN_Data]
  [Fan_NErr] -> NErr1/1
  Inlet/1 -> FAN/1, [S2]
  Pamb/1 -> [Pamb]
  Splitter_BPR/1 -> [Splitter_BPR]
  FAN/1 -> Fan_term2/1
  [Fan_Rline] -> FAN/2
  FAN/4 -> [Fan_NErr]
  duct2/1(GasPthCharOut) -> LPC/1, [S23]
  LPC/3 -> Valve/3
  LPC/6 -> [LPC_Data]
  LPC/1 -> LPC_term2/1
  LPC/2 -> LPC_term3/1
  LPC_Rline/1 -> [LPC_Rline]
  [LPC_Rline] -> LPC/2
  LPC/4 -> [LPC_NErr]
  [LPC_NErr] -> NErr2/1
  duct25/1(GasPthCharOut) -> [S25], FlwOut/1
  [LPC_TrqOut] -> LPC_Trq/1
  LP_Nmech/1 -> [LP_Nmech]
  [LP_Nmech] -> GearBox/2
  [LP_Nmech] -> LPC/3
  [S25] -> Bus Creator/8  "S25"
  [Fan_Nmech] -> Bus Creator/9  "N_Fan"
  [S24] -> Bus Creator/7  "S24"
  [S22] -> Bus Creator/5  "S22"
  [S23] -> Bus Creator/6  "S23"
  [S21] -> Bus Creator/3  "S21"
  [S2] -> Bus Creator/2  "S2"
  [S13] -> Bus Creator/4  "S13"
  [S0] -> Bus Creator/1  "S0"
  Bus Creator/1 -> F_Data/1
  AmbFlow/1 -> [S0], Inlet/1
  [Pamb] -> Inlet/2
  [LP_Nmech] -> Bus Creator/10  "N_LPC"
  [Fan_TrqGear] -> Bus Creator/11  "Trq_Fan"
  [LPC_TrqOut] -> Bus Creator/12  "Trq_LPC"
  LPC/5 -> [LPC_TrqOut]
  FAN/5 -> GearBox/1, [Fan_TrqGear]
  Valve/2 -> duct25/1(GasPthCharIn), [S24]
  Valve/1 -> BypFlow/1
  VBVdmd/1 -> [VBVdmd]
  [VBVdmd] -> Valve/2
  [VBVdmd] -> Bus Creator/13  "VBVdmd"
  [FAN_Data] -> Bus Creator/14  "FAN_Data"
  [LPC_Data] -> Bus Creator/15  "LPC_Data"
  Splitter/1 -> Valve/1, [S13]
  Valve/3 -> LPC_term1/1
  [LPC_Scalars] -> LPC/4
  LPC_Scalars/1 -> [LPC_Scalars]

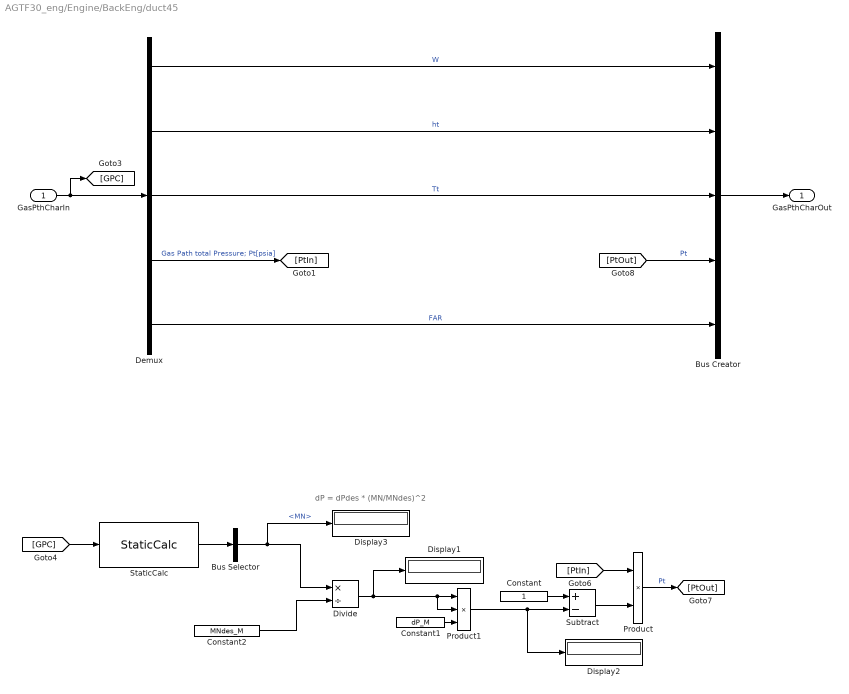
== system AGTF30_eng/Engine/BackEng/duct45 ==
  note: dP = dPdes * (MN/MNdes)^2
  GasPthCharIn : Inport
  Bus Selector : BusSelector  OutputSignals=MN
  Bus Creator : BusCreator  Inputs=5
  Constant : Constant
  Constant1 : Constant  Value=dP_M
  Constant2 : Constant  Value=MNdes_M
  Demux : Demux  Outputs=5
  Display1 : Display
  Display2 : Display
  Display3 : Display
  Divide : Product  Inputs=*/
  Product : Product  RndMeth=Zero
  Product1 : Product  Inputs=3  RndMeth=Zero
  StaticCalc : Lib_Turbo_StaticCalc_TMATS/StaticCalc  ST_M=off  Ath_M=Ath_M  MN_M=0.45  X_FARVec_M=[0; 0.0050; 0.0100; 0.0150; 0.0200; 0.0250; 0.0300]  Y_TtVec_M=[300 10000]  T_RtArray_M="[0.0686;    0.0686;    0.0686;    0.0686;    0.0686;    0.0686;    0.0686]"  T_gammaArray_M=[ 1.4 1.4 1.4 1.4 1.4 1.4 1.4; 1.4 1.4 1.4 1.4 1.4 1.4 1.4]
  Subtract : Sum  Inputs=+-
  GasPthCharOut : Outport
  wires:
  [GPC] -> StaticCalc/1
  Bus Selector/1 -> Divide/1, Display3/1  "<MN>"
  StaticCalc/1 -> Bus Selector/1
  Product/1 -> [PtOut]  "Pt"
  [PtIn] -> Product/1
  Product1/1 -> Subtract/2, Display2/1
  Divide/1 -> Product1/1, Product1/2, Display1/1
  Constant2/1 -> Divide/2
  Demux/2 -> Bus Creator/2  "ht"
  Subtract/1 -> Product/2
  Demux/4 -> [PtIn]  "Gas Path total Pressure; Pt[psia]"
  [PtOut] -> Bus Creator/4  "Pt"
  Bus Creator/1 -> GasPthCharOut/1
  GasPthCharIn/1 -> Demux/1, [GPC]
  Demux/3 -> Bus Creator/3  "Tt"
  Demux/5 -> Bus Creator/5  "FAR"
  Demux/1 -> Bus Creator/1  "W"
  Constant1/1 -> Product1/3
  Constant/1 -> Subtract/1

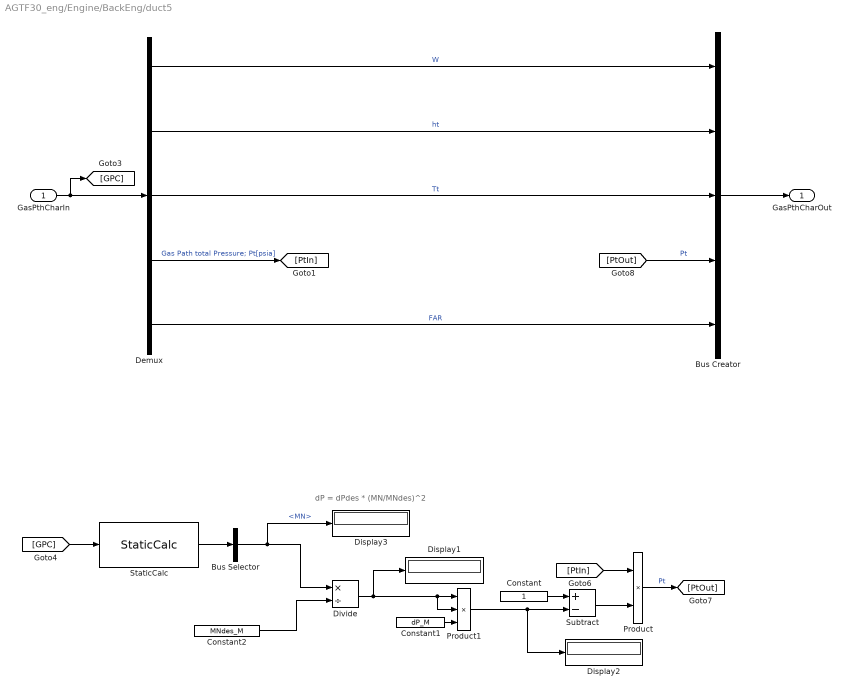
== system AGTF30_eng/Engine/BackEng/duct5 ==
  note: dP = dPdes * (MN/MNdes)^2
  GasPthCharIn : Inport
  Bus Selector : BusSelector  OutputSignals=MN
  Bus Creator : BusCreator  Inputs=5
  Constant : Constant
  Constant1 : Constant  Value=dP_M
  Constant2 : Constant  Value=MNdes_M
  Demux : Demux  Outputs=5
  Display1 : Display
  Display2 : Display
  Display3 : Display
  Divide : Product  Inputs=*/
  Product : Product  RndMeth=Zero
  Product1 : Product  Inputs=3  RndMeth=Zero
  StaticCalc : Lib_Turbo_StaticCalc_TMATS/StaticCalc  ST_M=off  Ath_M=Ath_M  MN_M=0.45  X_FARVec_M=[0; 0.0050; 0.0100; 0.0150; 0.0200; 0.0250; 0.0300]  Y_TtVec_M=[300 10000]  T_RtArray_M="[0.0686;    0.0686;    0.0686;    0.0686;    0.0686;    0.0686;    0.0686]"  T_gammaArray_M=[ 1.4 1.4 1.4 1.4 1.4 1.4 1.4; 1.4 1.4 1.4 1.4 1.4 1.4 1.4]
  Subtract : Sum  Inputs=+-
  GasPthCharOut : Outport
  wires:
  Constant/1 -> Subtract/1
  Constant1/1 -> Product1/3
  Demux/1 -> Bus Creator/1  "W"
  Demux/5 -> Bus Creator/5  "FAR"
  Demux/3 -> Bus Creator/3  "Tt"
  GasPthCharIn/1 -> [GPC], Demux/1
  Bus Creator/1 -> GasPthCharOut/1
  [PtOut] -> Bus Creator/4  "Pt"
  Demux/4 -> [PtIn]  "Gas Path total Pressure; Pt[psia]"
  Subtract/1 -> Product/2
  Demux/2 -> Bus Creator/2  "ht"
  Constant2/1 -> Divide/2
  Divide/1 -> Display1/1, Product1/2, Product1/1
  Product1/1 -> Display2/1, Subtract/2
  [PtIn] -> Product/1
  Product/1 -> [PtOut]  "Pt"
  StaticCalc/1 -> Bus Selector/1
  Bus Selector/1 -> Display3/1, Divide/1  "<MN>"
  [GPC] -> StaticCalc/1

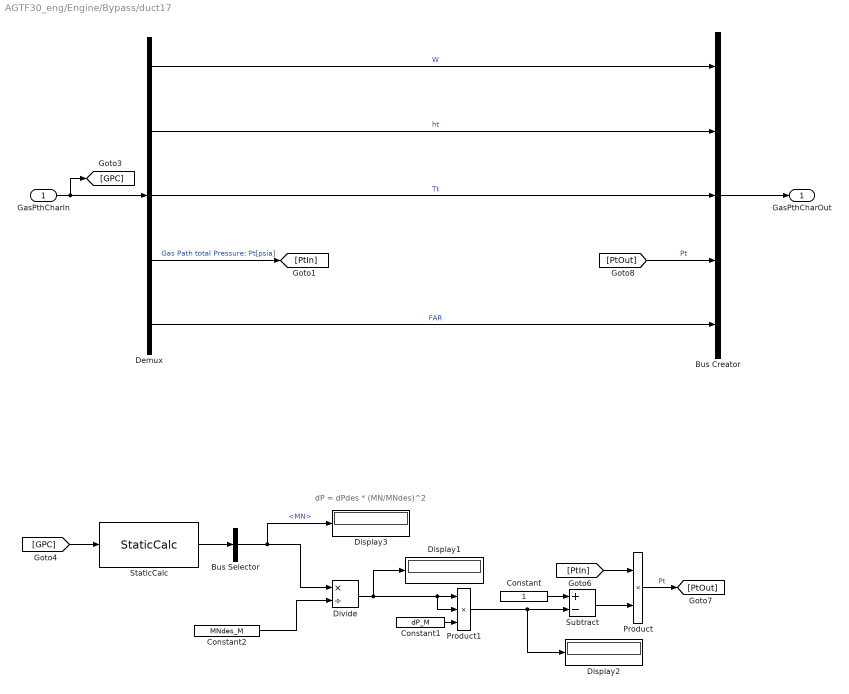
== system AGTF30_eng/Engine/Bypass/duct17 ==
  note: dP = dPdes * (MN/MNdes)^2
  GasPthCharIn : Inport
  Bus Selector : BusSelector  OutputSignals=MN
  Bus Creator : BusCreator  Inputs=5
  Constant : Constant
  Constant1 : Constant  Value=dP_M
  Constant2 : Constant  Value=MNdes_M
  Demux : Demux  Outputs=5
  Display1 : Display
  Display2 : Display
  Display3 : Display
  Divide : Product  Inputs=*/
  Product : Product  RndMeth=Zero
  Product1 : Product  Inputs=3  RndMeth=Zero
  StaticCalc : Lib_Turbo_StaticCalc_TMATS/StaticCalc  ST_M=off  Ath_M=Ath_M  MN_M=0.45  X_FARVec_M=[0; 0.0050; 0.0100; 0.0150; 0.0200; 0.0250; 0.0300]  Y_TtVec_M=[300 10000]  T_RtArray_M="[0.0686;    0.0686;    0.0686;    0.0686;    0.0686;    0.0686;    0.0686]"  T_gammaArray_M=[ 1.4 1.4 1.4 1.4 1.4 1.4 1.4; 1.4 1.4 1.4 1.4 1.4 1.4 1.4]
  Subtract : Sum  Inputs=+-
  GasPthCharOut : Outport
  wires:
  [GPC] -> StaticCalc/1
  Bus Selector/1 -> Divide/1, Display3/1  "<MN>"
  StaticCalc/1 -> Bus Selector/1
  Product/1 -> [PtOut]  "Pt"
  [PtIn] -> Product/1
  Product1/1 -> Subtract/2, Display2/1
  Divide/1 -> Product1/1, Product1/2, Display1/1
  Constant2/1 -> Divide/2
  Demux/2 -> Bus Creator/2  "ht"
  Subtract/1 -> Product/2
  Demux/4 -> [PtIn]  "Gas Path total Pressure; Pt[psia]"
  [PtOut] -> Bus Creator/4  "Pt"
  Bus Creator/1 -> GasPthCharOut/1
  GasPthCharIn/1 -> Demux/1, [GPC]
  Demux/3 -> Bus Creator/3  "Tt"
  Demux/5 -> Bus Creator/5  "FAR"
  Demux/1 -> Bus Creator/1  "W"
  Constant1/1 -> Product1/3
  Constant/1 -> Subtract/1

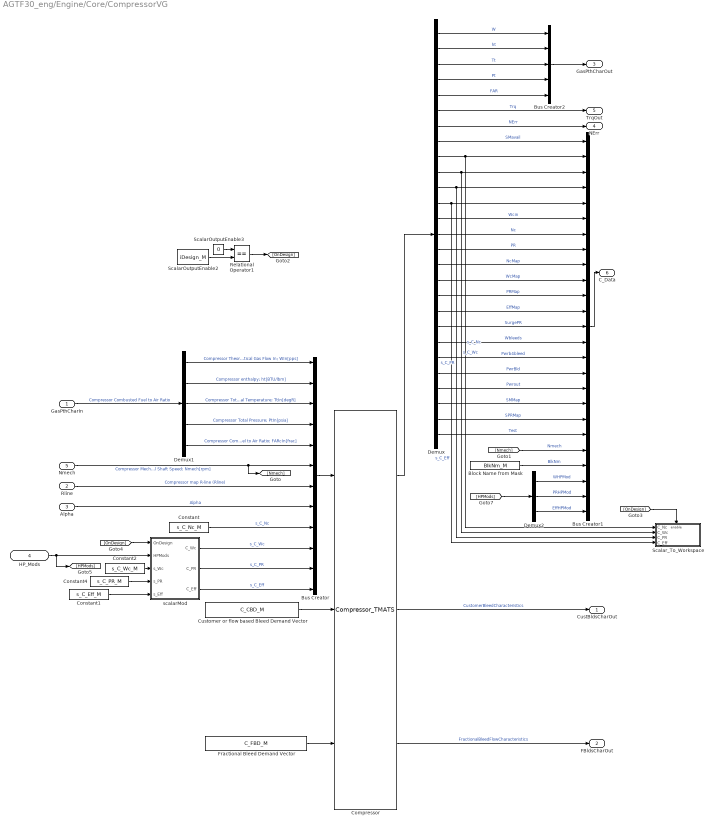
== system AGTF30_eng/Engine/Core/CompressorVG ==
  GasPthCharIn : Inport
  Rline : Inport  Port=2
  Alpha : Inport  Port=3
  HP_Mods : Inport  Port=4
  Nmech : Inport  Port=5
  Block Name from Mask : Constant  Value=BlkNm_M
  Bus Creator : BusCreator  Inputs=12
  Bus Creator1 : BusCreator  Inputs=25
  Bus Creator2 : BusCreator  Inputs=5
  Compressor : S-Function  FunctionName=Compressor_TMATS  Parameters="Y_C_Map_NcVec_M, X_C_RlineVec_M, Z_C_AlphaVec_M, T_C_Map_WcArray_M, T_C_Map_PRArray_M, T_C_Map_EffArray_M, C_CBFht_M, C_CBFPt_M,  C_BFht_M, C_BFPt_M, X_C_Map_WcSurgeVec_M, T_C_Map_PRSurgeVec_M, iDesign_M, SMNEn_M, NcDes_M, EffDes_M, PRDes_M, RlineDes_M, CBLDEN_M, FBLDEN_M, gcs, length(C_CBD_M), length(C_FBD_M), size(T_C_Map_WcArray_M,2), size(T_C_Map_PRArray_M,2), size(T_C_Map_EffArray_M,2), size(T_C_Map_WcArray_M,1), size(T_C_Map_PRArray_M,1), size(T_C_Map_EffArray_M,1), size(T_C_Map_WcArray_M,3), size(T_C_Map_PRArray_M,3), size(T_C_Map_EffArray_M,3)"  SFunctionModules='h2tc_TMATS pt2sc_TMATS sp2tc_TMATS t2hc_TMATS interp1Ac_TMATS interp2Ac_TMATS interp3Ac_TMATS functions_TMATS'
  Constant : Constant  Value=s_C_Nc_M
  Constant1 : Constant  Value=s_C_Eff_M
  Constant2 : Constant  Value=s_C_Wc_M
  Constant4 : Constant  Value=s_C_PR_M
  Customer or flow based Bleed Demand Vector : Constant  Value=C_CBD_M
  Demux : Demux  Outputs=27
  Demux1 : Demux  Outputs=5
  Demux2 : Demux  Outputs=3
  Fractional Bleed Demand Vector : Constant  Value=C_FBD_M
  Relational Operator1 : RelationalOperator  Operator===  OutDataTypeStr=boolean
  ScalarOutputEnable2 : Constant  Value=iDesign_M
  ScalarOutputEnable3 : Constant  Value=0
  Scalar_To_Workspace : Subsystem
  scalarMod : Subsystem
  CustBldsCharOut : Outport  PortDimensions=length(C_CBD_M)*5
  FBldsCharOut : Outport  Port=2  PortDimensions=length(C_FBD_M)*5
  GasPthCharOut : Outport  Port=3
  NErr : Outport  Port=4
  TrqOut : Outport  Port=5
  C_Data : Outport  Port=6
  wires:
  Demux2/3 -> Bus Creator1/25  "EffHPMod"
  Demux2/2 -> Bus Creator1/24  "PRHPMod"
  Demux2/1 -> Bus Creator1/23  "WHPMod"
  [HPMods] -> Demux2/1
  HP_Mods/1 -> scalarMod/2(HPMods), [HPMods]
  [OnDesign] -> scalarMod/1(OnDesign)
  Constant1/1 -> scalarMod/5(s_Eff)
  Constant4/1 -> scalarMod/4(s_PR)
  Constant2/1 -> scalarMod/3(s_Wc)
  [OnDesign] -> Scalar_To_Workspace/Enable
  Relational Operator1/1 -> [OnDesign]
  ScalarOutputEnable3/1 -> Relational Operator1/1
  ScalarOutputEnable2/1 -> Relational Operator1/2
  Alpha/1 -> Bus Creator/8  "Alpha"
  Constant/1 -> Bus Creator/9  "s_C_Nc"
  scalarMod/2(C_PR) -> Bus Creator/11  "s_C_PR"
  scalarMod/1(C_Wc) -> Bus Creator/10  "s_C_Wc"
  scalarMod/3(C_Eff) -> Bus Creator/12  "s_C_Eff"
  Block Name from Mask/1 -> Bus Creator1/22  "BlkNm"
  [Nmech] -> Bus Creator1/21  "Nmech"
  Demux/27 -> Bus Creator1/20  "Test"
  Demux/26 -> Bus Creator1/19  "SPRMap"
  Demux/25 -> Bus Creator1/18  "SMMap"
  Demux/18 -> Bus Creator1/11  "PRMap"
  Demux/15 -> Bus Creator1/8  "PR"
  Demux/17 -> Bus Creator1/10  "WcMap"
  Demux/19 -> Bus Creator1/12  "EffMap"
  Demux/24 -> Bus Creator1/17  "Pwrout"
  Demux/16 -> Bus Creator1/9  "NcMap"
  Demux/20 -> Bus Creator1/13  "SurgePR"
  Demux/21 -> Bus Creator1/14  "Wbleeds"
  Demux/22 -> Bus Creator1/15  "Pwrb4bleed"
  Demux/23 -> Bus Creator1/16  "PwrBld"
  Demux/14 -> Bus Creator1/7  "Nc"
  Demux/12 -> Bus Creator1/5, Scalar_To_Workspace/4(C_Eff)  "s_C_Eff"
  Demux/11 -> Bus Creator1/4, Scalar_To_Workspace/3(C_PR)  "s_C_PR"
  Demux/10 -> Bus Creator1/3, Scalar_To_Workspace/2(C_Wc)  "s_C_Wc"
  Demux/9 -> Bus Creator1/2, Scalar_To_Workspace/1(C_Nc)  "s_C_Nc"
  Bus Creator1/1 -> C_Data/1
  Demux/8 -> Bus Creator1/1  "SMavail"
  Demux1/2 -> Bus Creator/2  "Compressor enthalpy; ht[BTU/lbm]"
  Compressor/3 -> FBldsCharOut/1  "FractionalBleedFlowCharacteristics"
  Compressor/2 -> CustBldsCharOut/1  "CustomerBleedCharacteristics"
  Fractional Bleed Demand Vector/1 -> Compressor/3
  Customer or flow based Bleed Demand Vector/1 -> Compressor/2
  Demux/7 -> NErr/1  "NErr"
  Demux1/1 -> Bus Creator/1  "Compressor Theoretical Gas Flow In; WIn[pps]"
  GasPthCharIn/1 -> Demux1/1  "Compressor Combusted Fuel to Air Ratio"
  Bus Creator2/1 -> GasPthCharOut/1
  Demux/2 -> Bus Creator2/2  "ht"
  Demux/13 -> Bus Creator1/6  "Wcin"
  Rline/1 -> Bus Creator/7  "Compressor map R-line (Rline)"
  Demux1/5 -> Bus Creator/5  "Compressor Combusted Fuel to Air Ratio; FARcIn[frac]"
  Demux1/3 -> Bus Creator/3  "Compressor Total Temperature; TtIn[degR]"
  Compressor/1 -> Demux/1
  Demux/1 -> Bus Creator2/1  "W"
  Demux/5 -> Bus Creator2/5  "FAR"
  Demux/3 -> Bus Creator2/3  "Tt"
  Demux/4 -> Bus Creator2/4  "Pt"
  Bus Creator/1 -> Compressor/1
  Demux/6 -> TrqOut/1  "Trq"
  Nmech/1 -> Bus Creator/6, [Nmech]  "Compressor Mechanical Shaft Speed; Nmech[rpm]"
  Demux1/4 -> Bus Creator/4  "Compressor Total Pressure; PtIn[psia]"

== system AGTF30_eng/Engine/Core/S36 Static Calc ==
  S36t : Inport
  Bus Selector2 : BusSelector  OutputSignals=W,ht,Tt,Pt,FAR
  Mux4 : Mux  Inputs=5
  StaticCalc : Lib_Turbo_StaticCalc_TMATS/StaticCalc  ST_M=off  Ath_M=MWS.HPC.Ath  MN_M=0.3  X_FARVec_M=[0; 0.0050; 0.0100; 0.0150; 0.0200; 0.0250; 0.0300]  Y_TtVec_M=[300 10000]  T_RtArray_M="[0.0686;    0.0686;    0.0686;    0.0686;    0.0686;    0.0686;    0.0686]"  T_gammaArray_M=[ 1.4 1.4 1.4 1.4 1.4 1.4 1.4; 1.4 1.4 1.4 1.4 1.4 1.4 1.4]
  S36stc : Outport
  wires:
  Bus Selector2/4 -> Mux4/4  "<Pt>"
  Bus Selector2/2 -> Mux4/2  "<ht>"
  Bus Selector2/5 -> Mux4/5  "<FAR>"
  Bus Selector2/1 -> Mux4/1  "<W>"
  Bus Selector2/3 -> Mux4/3  "<Tt>"
  Mux4/1 -> StaticCalc/1
  StaticCalc/1 -> S36stc/1
  S36t/1 -> Bus Selector2/1

== system AGTF30_eng/Engine/Core/S36bus ==
  S36tot : Inport
  S36stat : Inport  Port=2
  Bus Creator1 : BusCreator  Inputs=7
  Bus Selector : BusSelector  OutputSignals=Ps,Ts
  Bus Selector1 : BusSelector  OutputSignals=W,ht,Tt,Pt,FAR
  S36all : Outport
  wires:
  Bus Selector1/2 -> Bus Creator1/2  "<ht>"
  Bus Selector1/1 -> Bus Creator1/1  "<W>"
  Bus Selector1/5 -> Bus Creator1/5  "<FAR>"
  Bus Selector/2 -> Bus Creator1/7  "<Ts>"
  S36stat/1 -> Bus Selector/1
  S36tot/1 -> Bus Selector1/1
  Bus Selector/1 -> Bus Creator1/6  "<Ps>"
  Bus Creator1/1 -> S36all/1
  Bus Selector1/3 -> Bus Creator1/3  "<Tt>"
  Bus Selector1/4 -> Bus Creator1/4  "<Pt>"

== system AGTF30_eng/Engine/EngData/CompressorSurgeMargin ==
  Front : Inport
  Core : Inport  Port=2
  Bus Creator : BusCreator  Inputs=3
  Bus Selector6 : BusSelector  OutputSignals=HPC_Data.SMMap
  Bus Selector7 : BusSelector  OutputSignals=FAN_Data.SMMap,LPC_Data.SMMap
  Gain : Gain
  Gain1 : Gain
  Gain2 : Gain
  SM : Outport
  wires:
  Bus Selector6/1 -> Gain2/1  "<SMMap>"
  Core/1 -> Bus Selector6/1
  Gain2/1 -> Bus Creator/3  "SMHPC"
  Bus Selector7/1 -> Gain/1  "<SMMap>"
  Bus Selector7/2 -> Gain1/1  "<SMMap>"
  Front/1 -> Bus Selector7/1
  Gain/1 -> Bus Creator/1  "SMFan"
  Gain1/1 -> Bus Creator/2  "SMLPC"
  Bus Creator/1 -> SM/1

== system AGTF30_eng/Engine/EngData/CompressorTurbineDataBus ==
  Front : Inport
  Core : Inport  Port=2
  Back : Inport  Port=3
  Bus Creator : BusCreator  Inputs=5
  Bus Selector10 : BusSelector  OutputSignals=LPT_Data
  Bus Selector8 : BusSelector  OutputSignals=FAN_Data,LPC_Data
  Bus Selector9 : BusSelector  OutputSignals=HPC_Data,HPT_Data
  Data : Outport
  wires:
  Bus Selector8/1 -> Bus Creator/1  "<FAN_Data>"
  Bus Selector10/1 -> Bus Creator/5  "<LPT_Data>"
  Front/1 -> Bus Selector8/1
  Bus Selector8/2 -> Bus Creator/2  "<LPC_Data>"
  Back/1 -> Bus Selector10/1
  Bus Selector9/2 -> Bus Creator/4  "<HPT_Data>"
  Bus Creator/1 -> Data/1
  Bus Selector9/1 -> Bus Creator/3  "<HPC_Data>"
  Core/1 -> Bus Selector9/1

== system AGTF30_eng/Engine/EngData/Performance ==
  Front : Inport
  Core : Inport  Port=2
  Bypass : Inport  Port=3
  Fg : Inport  Port=4
  Fnet : Inport  Port=5
  TSFC : Inport  Port=6
  Bus Creator : BusCreator  Inputs=6
  Bus Selector1 : BusSelector  OutputSignals=Fg_Core
  Bus Selector2 : BusSelector  OutputSignals=Fg_Byp
  Bus Selector3 : BusSelector  OutputSignals=Fdrag
  Performance : Outport
  wires:
  Fnet/1 -> Bus Creator/5  "Fnet"
  Bus Selector2/1 -> Bus Creator/3  "<Fg_Byp>"
  Bus Selector3/1 -> Bus Creator/1  "<Fdrag>"
  Front/1 -> Bus Selector3/1
  Bypass/1 -> Bus Selector2/1
  Core/1 -> Bus Selector1/1
  Bus Selector1/1 -> Bus Creator/2  "<Fg_Core>"
  Fg/1 -> Bus Creator/4  "Fg"
  Bus Creator/1 -> Performance/1
  TSFC/1 -> Bus Creator/6  "TSFC"

== system AGTF30_eng/Engine/EngData/Shafts ==
  Front : Inport
  Core : Inport  Port=2
  Ndot_LP : Inport  Port=3
  Ndot_HP : Inport  Port=4
  Bus Creator : BusCreator  Inputs=5
  Bus Selector4 : BusSelector  OutputSignals=N_Fan,N_LPC
  Bus Selector5 : BusSelector  OutputSignals=N_HPC
  Shaft : Outport
  wires:
  Front/1 -> Bus Selector4/1
  Bus Selector5/1 -> Bus Creator/3  "<N_HPC>"
  Bus Selector4/1 -> Bus Creator/1  "<N_Fan>"
  Core/1 -> Bus Selector5/1
  Bus Selector4/2 -> Bus Creator/2  "<N_LPC>"
  Ndot_LP/1 -> Bus Creator/4  "Ndot_LPC"
  Ndot_HP/1 -> Bus Creator/5  "Ndot_HPC"
  Bus Creator/1 -> Shaft/1

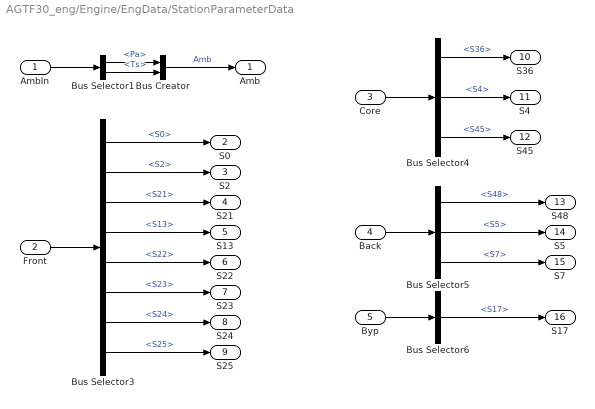
== system AGTF30_eng/Engine/EngData/StationParameterData ==
  AmbIn : Inport
  Front : Inport  Port=2
  Core : Inport  Port=3
  Back : Inport  Port=4
  Byp : Inport  Port=5
  Bus Creator : BusCreator  Inputs=2
  Bus Selector1 : BusSelector  OutputSignals=Pa,Ts
  Bus Selector3 : BusSelector  OutputSignals=S0,S2,S21,S13,S22,S23,S24,S25
  Bus Selector4 : BusSelector  OutputSignals=S36,S4,S45
  Bus Selector5 : BusSelector  OutputSignals=S48,S5,S7
  Bus Selector6 : BusSelector  OutputSignals=S17
  Amb : Outport
  S0 : Outport  Port=2
  S2 : Outport  Port=3
  S21 : Outport  Port=4
  S13 : Outport  Port=5
  S22 : Outport  Port=6
  S23 : Outport  Port=7
  S24 : Outport  Port=8
  S25 : Outport  Port=9
  S36 : Outport  Port=10
  S4 : Outport  Port=11
  S45 : Outport  Port=12
  S48 : Outport  Port=13
  S5 : Outport  Port=14
  S7 : Outport  Port=15
  S17 : Outport  Port=16
  wires:
  Back/1 -> Bus Selector5/1
  Bus Selector3/7 -> S24/1  "<S24>"
  Bus Selector3/4 -> S13/1  "<S13>"
  Bus Selector5/2 -> S5/1  "<S5>"
  Bus Selector1/2 -> Bus Creator/2  "<Ts>"
  Bus Selector5/1 -> S48/1  "<S48>"
  Bus Selector4/2 -> S4/1  "<S4>"
  Bus Creator/1 -> Amb/1  "Amb"
  Bus Selector3/5 -> S22/1  "<S22>"
  Bus Selector1/1 -> Bus Creator/1  "<Pa>"
  Bus Selector5/3 -> S7/1  "<S7>"
  Core/1 -> Bus Selector4/1
  Bus Selector6/1 -> S17/1  "<S17>"
  Bus Selector3/8 -> S25/1  "<S25>"
  Bus Selector4/3 -> S45/1  "<S45>"
  Bus Selector3/3 -> S21/1  "<S21>"
  Front/1 -> Bus Selector3/1
  AmbIn/1 -> Bus Selector1/1
  Bus Selector3/2 -> S2/1  "<S2>"
  Bus Selector3/1 -> S0/1  "<S0>"
  Byp/1 -> Bus Selector6/1
  Bus Selector3/6 -> S23/1  "<S23>"
  Bus Selector4/1 -> S36/1  "<S36>"

== system AGTF30_eng/Engine/FrontEng/duct2 ==
  note: dP = dPdes * (MN/MNdes)^2
  GasPthCharIn : Inport
  Bus Selector : BusSelector  OutputSignals=MN
  Bus Creator : BusCreator  Inputs=5
  Constant : Constant
  Constant1 : Constant  Value=dP_M
  Constant2 : Constant  Value=MNdes_M
  Demux : Demux  Outputs=5
  Display1 : Display
  Display2 : Display
  Display3 : Display
  Divide : Product  Inputs=*/
  Product : Product  RndMeth=Zero
  Product1 : Product  Inputs=3  RndMeth=Zero
  StaticCalc : Lib_Turbo_StaticCalc_TMATS/StaticCalc  ST_M=off  Ath_M=Ath_M  MN_M=0.45  X_FARVec_M=[0; 0.0050; 0.0100; 0.0150; 0.0200; 0.0250; 0.0300]  Y_TtVec_M=[300 10000]  T_RtArray_M="[0.0686;    0.0686;    0.0686;    0.0686;    0.0686;    0.0686;    0.0686]"  T_gammaArray_M=[ 1.4 1.4 1.4 1.4 1.4 1.4 1.4; 1.4 1.4 1.4 1.4 1.4 1.4 1.4]
  Subtract : Sum  Inputs=+-
  GasPthCharOut : Outport
  wires:
  Constant/1 -> Subtract/1
  Constant1/1 -> Product1/3
  Demux/1 -> Bus Creator/1  "W"
  Demux/5 -> Bus Creator/5  "FAR"
  Demux/3 -> Bus Creator/3  "Tt"
  GasPthCharIn/1 -> [GPC], Demux/1
  Bus Creator/1 -> GasPthCharOut/1
  [PtOut] -> Bus Creator/4  "Pt"
  Demux/4 -> [PtIn]  "Gas Path total Pressure; Pt[psia]"
  Subtract/1 -> Product/2
  Demux/2 -> Bus Creator/2  "ht"
  Constant2/1 -> Divide/2
  Divide/1 -> Display1/1, Product1/2, Product1/1
  Product1/1 -> Display2/1, Subtract/2
  [PtIn] -> Product/1
  Product/1 -> [PtOut]  "Pt"
  StaticCalc/1 -> Bus Selector/1
  Bus Selector/1 -> Display3/1, Divide/1  "<MN>"
  [GPC] -> StaticCalc/1

== system AGTF30_eng/Engine/FrontEng/duct25 ==
  note: dP = dPdes * (MN/MNdes)^2
  GasPthCharIn : Inport
  Bus Selector : BusSelector  OutputSignals=MN
  Bus Creator : BusCreator  Inputs=5
  Constant : Constant
  Constant1 : Constant  Value=dP_M
  Constant2 : Constant  Value=MNdes_M
  Demux : Demux  Outputs=5
  Display1 : Display
  Display2 : Display
  Display3 : Display
  Divide : Product  Inputs=*/
  Product : Product  RndMeth=Zero
  Product1 : Product  Inputs=3  RndMeth=Zero
  StaticCalc : Lib_Turbo_StaticCalc_TMATS/StaticCalc  ST_M=off  Ath_M=Ath_M  MN_M=0.45  X_FARVec_M=[0; 0.0050; 0.0100; 0.0150; 0.0200; 0.0250; 0.0300]  Y_TtVec_M=[300 10000]  T_RtArray_M="[0.0686;    0.0686;    0.0686;    0.0686;    0.0686;    0.0686;    0.0686]"  T_gammaArray_M=[ 1.4 1.4 1.4 1.4 1.4 1.4 1.4; 1.4 1.4 1.4 1.4 1.4 1.4 1.4]
  Subtract : Sum  Inputs=+-
  GasPthCharOut : Outport
  wires:
  [GPC] -> StaticCalc/1
  Bus Selector/1 -> Divide/1, Display3/1  "<MN>"
  StaticCalc/1 -> Bus Selector/1
  Product/1 -> [PtOut]  "Pt"
  [PtIn] -> Product/1
  Product1/1 -> Subtract/2, Display2/1
  Divide/1 -> Product1/1, Product1/2, Display1/1
  Constant2/1 -> Divide/2
  Demux/2 -> Bus Creator/2  "ht"
  Subtract/1 -> Product/2
  Demux/4 -> [PtIn]  "Gas Path total Pressure; Pt[psia]"
  [PtOut] -> Bus Creator/4  "Pt"
  Bus Creator/1 -> GasPthCharOut/1
  GasPthCharIn/1 -> Demux/1, [GPC]
  Demux/3 -> Bus Creator/3  "Tt"
  Demux/5 -> Bus Creator/5  "FAR"
  Demux/1 -> Bus Creator/1  "W"
  Constant1/1 -> Product1/3
  Constant/1 -> Subtract/1

== system AGTF30_eng/Engine/Core/CompressorVG/Scalar_To_Workspace ==
  C_Nc : Inport
  C_Wc : Inport  Port=2
  C_PR : Inport  Port=3
  C_Eff : Inport  Port=4
  Enable : EnablePort
  DataOutput : Lib_Solve_DataOut_TMATS/DataOutput  FVar_M=double(FVar_M)
  Mux : Mux
  wires:
  Mux/1 -> DataOutput/1
  C_Eff/1 -> Mux/4
  C_PR/1 -> Mux/3
  C_Wc/1 -> Mux/2
  C_Nc/1 -> Mux/1

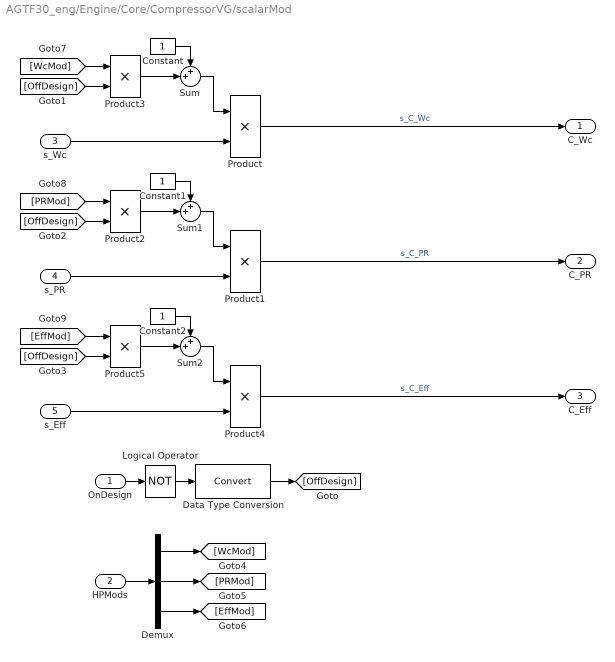
== system AGTF30_eng/Engine/Core/CompressorVG/scalarMod ==
  OnDesign : Inport
  HPMods : Inport  Port=2
  s_Wc : Inport  Port=3
  s_PR : Inport  Port=4
  s_Eff : Inport  Port=5
  Constant : Constant
  Constant1 : Constant
  Constant2 : Constant
  Data Type Conversion : DataTypeConversion
  Demux : Demux  Outputs=3
  Logical Operator : Logic  Operator=NOT  AllPortsSameDT=off  OutDataTypeStr=boolean
  Product{,1..5} (6 alike) : Product
  Sum : Sum  Inputs=++|
  Sum1 : Sum  Inputs=++|
  Sum2 : Sum  Inputs=++|
  C_Wc : Outport
  C_PR : Outport  Port=2
  C_Eff : Outport  Port=3
  wires:
  Product1/1 -> C_PR/1  "s_C_PR"
  Product4/1 -> C_Eff/1  "s_C_Eff"
  Product/1 -> C_Wc/1  "s_C_Wc"
  s_Wc/1 -> Product/2
  OnDesign/1 -> Logical Operator/1
  Data Type Conversion/1 -> [OffDesign]
  Logical Operator/1 -> Data Type Conversion/1
  Sum/1 -> Product/1
  [WcMod] -> Product3/1
  Constant/1 -> Sum/1
  Product3/1 -> Sum/2
  [OffDesign] -> Product3/2
  s_PR/1 -> Product1/2
  Sum1/1 -> Product1/1
  [PRMod] -> Product2/1
  Constant1/1 -> Sum1/1
  Product2/1 -> Sum1/2
  [OffDesign] -> Product2/2
  s_Eff/1 -> Product4/2
  Sum2/1 -> Product4/1
  [EffMod] -> Product5/1
  Constant2/1 -> Sum2/1
  Product5/1 -> Sum2/2
  [OffDesign] -> Product5/2
  HPMods/1 -> Demux/1
  Demux/1 -> [WcMod]
  Demux/2 -> [PRMod]
  Demux/3 -> [EffMod]
